simulink model "SimuModel_H_robust"  (Simulink 9.3)
settings: Solver=ode23  StartTime=0.0  StopTime=t_d  MaxStep=Tc  RelTol=1e-8  AbsTol=1e-8
values from neighbouring files (symbols this model uses):
  B_h = diag([a(1)*pi_l(1) + pi_l(2) + a(2) + pi_l(4) ... (first row only)    [InitVariable_exe.m]
  DQ = D'*Q    [InitVariable_exe.m]
  ep = 0.004    [InitVariable_exe.m]
  F_v = K_r*diag([0.01 0.01])*K_r    [InitVariable_exe.m]
  g = 9.81    [InitVariable_exe.m]
  K_d = 5*diag([1 1])    [InitVariable_exe.m]
  K_p = 25*diag([1 1])    [InitVariable_exe.m]
  q_i = [-1.4706; 2.9413]    [InitVariable_exe.m]
  rho = 70    [InitVariable_exe.m]
  Tc = 0.001    [InitVariable_exe.m]
  Ts = Tc    (= 0.001)    [InitVariable_exe.m]
undefined symbols (not defined in the file or in its folder): a, BMatrix, pi_l, pi_m
settings Model: Creator=luigivillani  LastModifiedBy=yuzg  ExtModeAutoUpdateStatusClock=off
settings SolverCC: AutoScaleAbsTol=off  InitialStep=0.1*Tc
settings DataIOCC: SaveOutput=off  SaveTime=off
settings OptimizationCC: BlockReduction=off  BooleanDataType=off  ExpressionDepthLimit=2147483647  InitFltsAndDblsToZero=on
settings DebuggingCC: SaveWithParameterizedLinksMsg=none  SignalResolutionControl=TryResolveAllWithWarning  MultiTaskDSMMsg=warning  MultiTaskCondExecSysMsg=none  StateNameClashWarn=warning
settings HardwareCC: TargetUnknown=on
settings SFSimCC: SimUseLocalCustomCode=on
settings RTWCC: RTWUseLocalCustomCode=on
settings GRTTargetCC: TargetFcnLib=ansi_tfl_tmw.mat
settings ConfigComp: CovExternalEMLEnable=on

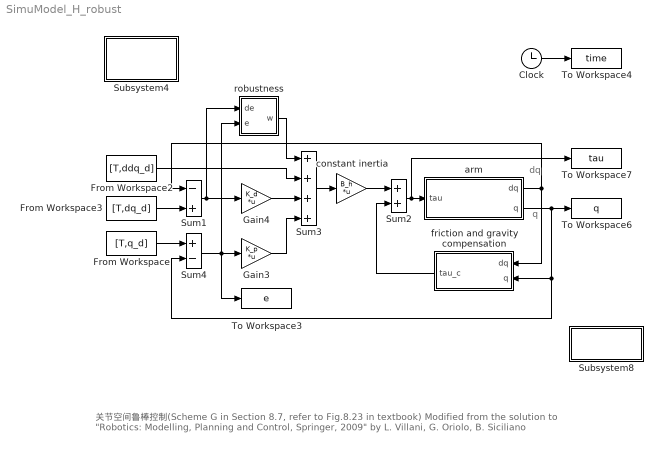
== system SimuModel_H_robust ==
  note: dq
  note: q
  note: 关节空间鲁棒控制(Scheme G in Section 8.7, refer to Fig.8.23 in textbook)
      | Modified from the solution to "Robotics: Modelling, Planning and Control, Springer, 2009" by L. Villani, G. Oriolo, B. Siciliano
  Clock : Clock
  From Workspace : FromWorkspace  VariableName=[T,q_d]  SampleTime=Tc
  From Workspace2 : FromWorkspace  VariableName=[T,ddq_d]  SampleTime=Tc
  From Workspace3 : FromWorkspace  VariableName=[T,dq_d]  SampleTime=Tc
  Gain3 : Gain  Gain=K_p  Multiplication=Matrix(K*u)  SampleTime=Tc
      mask Display: disp('K_p')
  Gain4 : Gain  Gain=K_d  Multiplication=Matrix(K*u)  SampleTime=Tc
      mask Display: disp('K_d')
  Subsystem4 : Subsystem
      settings: OpenFcn=clear all;c=0;InitVariable_exe;
      mask Display: disp('K_p = 25I\nK_d = 5I')
  Subsystem8 : Subsystem
      settings: OpenFcn=PlotFigure;
      mask Display: disp('plot')
  Sum1 : Sum  Inputs=-+  SampleTime=Tc  SaturateOnIntegerOverflow=on  InputSameDT=on  OutDataTypeStr=Inherit: Same as first input
  Sum2 : Sum  SaturateOnIntegerOverflow=on  InputSameDT=on  OutDataTypeStr=Inherit: Same as first input
  Sum3 : Sum  Inputs=++++  SaturateOnIntegerOverflow=on  InputSameDT=on  OutDataTypeStr=Inherit: Same as first input
  Sum4 : Sum  Inputs=+-  SampleTime=Tc  SaturateOnIntegerOverflow=on  InputSameDT=on  OutDataTypeStr=Inherit: Same as first input
  To Workspace3 : ToWorkspace  VariableName=e  SampleTime=Ts
      settings: MaxDataPoints=5001
  To Workspace4 : ToWorkspace  VariableName=time  SampleTime=Ts
      settings: MaxDataPoints=5001
  To Workspace6 : ToWorkspace  VariableName=q  SampleTime=Ts
      settings: MaxDataPoints=5001
  To Workspace7 : ToWorkspace  VariableName=tau  SampleTime=Ts
      settings: MaxDataPoints=5001
  arm : Subsystem
      mask Display: disp('Robot InvDynamics')
  constant inertia : Gain  Gain=B_h  Multiplication=Matrix(K*u)  SampleTime=Tc
      mask Display: disp('B_h')
  friction and gravity compensation : Subsystem
      mask Display: disp('F_vdq+g(q)')
  robustness : Subsystem
      mask Display: disp('UV')
  wires:
  Clock/1 -> To Workspace4/1
  Sum3/1 -> constant inertia/1
  friction and gravity compensation/1(tau_c) -> Sum2/2
  arm/1(dq) -> Sum1/1, friction and gravity compensation/1(dq)
  arm/2("q ") -> To Workspace6/1, friction and gravity compensation/2(q), Sum4/2
  From Workspace3/1 -> Sum1/2
  From Workspace/1 -> Sum4/1
  constant inertia/1 -> Sum2/1
  Sum4/1 -> robustness/2(e), To Workspace3/1, Gain3/1
  Sum1/1 -> robustness/1(de), Gain4/1
  Gain3/1 -> Sum3/4
  Gain4/1 -> Sum3/3
  Sum2/1 -> To Workspace7/1, arm/1(tau)
  robustness/1(w) -> Sum3/1
  From Workspace2/1 -> Sum3/2

== system SimuModel_H_robust/Subsystem4 ==
  note: start

== system SimuModel_H_robust/Subsystem8 ==
  note: start

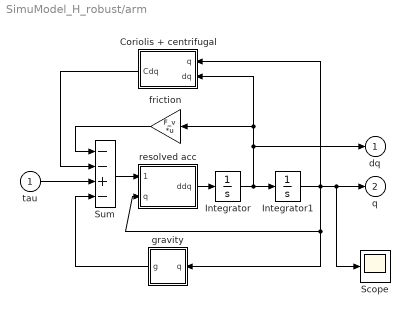
== system SimuModel_H_robust/arm ==
  tau : Inport
  Coriolis + centrifugal : Subsystem
      mask Display: disp('C(q,dq)dq')
  Integrator : Integrator  InitialCondition=[0 0]  ZeroCross=off
  Integrator1 : Integrator  InitialCondition=q_i  ZeroCross=off
  Scope : Scope
  Sum : Sum  Inputs=--+-  SaturateOnIntegerOverflow=on  InputSameDT=on  OutDataTypeStr=Inherit: Same as first input
  friction : Gain  Gain=F_v  Multiplication=Matrix(K*u)  SaturateOnIntegerOverflow=on  OutDataTypeStr=Inherit: Same as input  ParamDataTypeStr=Inherit: Same as input
      mask Display: disp('F_v')
  gravity : Subsystem
      mask Display: disp('g(q)')
  resolved acc : Subsystem
      mask Display: disp('inv(B(q))')
  dq : Outport  InitialOutput=0
  "q " : Outport  Port=2  InitialOutput=0
  wires:
  Coriolis + centrifugal/1(Cdq) -> Sum/2
  tau/1 -> Sum/3
  Integrator1/1 -> Coriolis + centrifugal/1(q), resolved acc/2(q), gravity/1(q), Scope/1, "q "/1
  resolved acc/1(ddq) -> Integrator/1
  Integrator/1 -> Integrator1/1, dq/1, Coriolis + centrifugal/2(dq), friction/1
  Sum/1 -> resolved acc/1(tau-tau')
  friction/1 -> Sum/1
  gravity/1(g) -> Sum/4

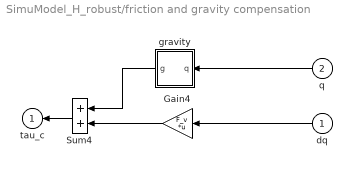
== system SimuModel_H_robust/friction and gravity compensation ==
  dq : Inport
  q : Inport  Port=2
  Gain4 : Gain  Gain=F_v  Multiplication=Matrix(K*u)  SampleTime=Tc
      mask Display: disp('F_v')
  Sum4 : Sum  SaturateOnIntegerOverflow=on  InputSameDT=on  OutDataTypeStr=Inherit: Same as first input
  gravity : Subsystem
      mask Display: disp('g(q)')
  tau_c : Outport  InitialOutput=0
  wires:
  gravity/1(g) -> Sum4/1
  Sum4/1 -> tau_c/1
  q/1 -> gravity/1(q)
  Gain4/1 -> Sum4/2
  dq/1 -> Gain4/1

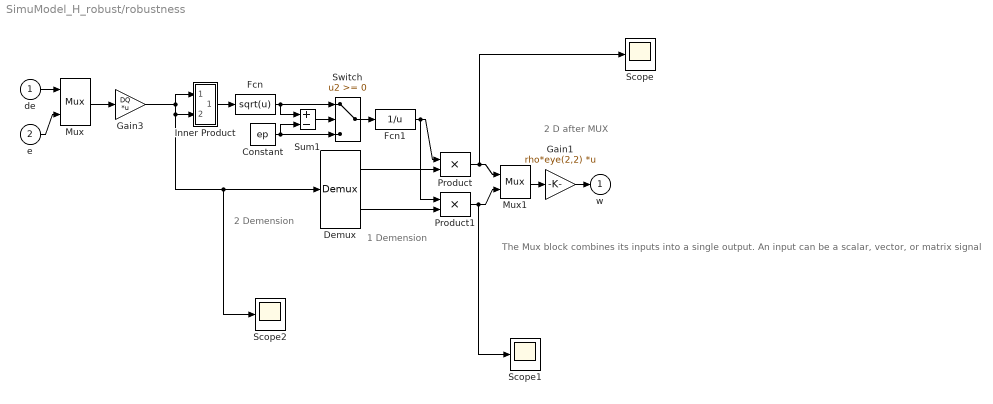
== system SimuModel_H_robust/robustness ==
  note: 2 Demension
  note: The Mux block combines its inputs into a single output. An input can be a scalar, vector, or matrix signal
  note: 1 Demension
  note: 2 D after MUX
  de : Inport
  e : Inport  Port=2
  Constant : Constant  Value=ep
  Demux : Demux  Outputs=2
  Fcn : Fcn  Expr=sqrt(u)
  Fcn1 : Fcn  Expr=1/u  SampleTime=Tc
  Gain1 : Gain  Gain=rho*eye(2,2)  Multiplication=Matrix(K*u)  SampleTime=Tc
      mask Display: disp('rho')
  Gain3 : Gain  Gain=DQ  Multiplication=Matrix(K*u)  SampleTime=Tc
      mask Display: disp('DQ')
  Inner Product : Subsystem  mask(Dot Product){}
      mask help:
      | Inner (dot) product.
      | y=sum(u1.*u2)
      mask Help: Computes the inner (dot) product of the inputs: sum(u1.*u2).  The inputs are vectors of the same length. Output is a scalar.
      mask Display: disp('.\n')
  Mux : Mux  Inputs=[2,2]
  Mux1 : Mux  Inputs=2
  Product : Product  SaturateOnIntegerOverflow=on  RndMeth=Zero  InputSameDT=on  OutDataTypeStr=Inherit: Same as first input
  Product1 : Product  SaturateOnIntegerOverflow=on  RndMeth=Zero  InputSameDT=on  OutDataTypeStr=Inherit: Same as first input
  Scope : Scope
  Scope1 : Scope
  Scope2 : Scope
  Sum1 : Sum  Inputs=+-  SaturateOnIntegerOverflow=on  InputSameDT=on  OutDataTypeStr=Inherit: Same as first input
  Switch : Switch  SaturateOnIntegerOverflow=on  InputSameDT=on
  w : Outport  InitialOutput=0
  wires:
  Demux/2 -> Product1/2
  Demux/1 -> Product/2
  Product1/1 -> Scope1/1, Mux1/2
  Product/1 -> Scope/1, Mux1/1
  Switch/1 -> Fcn1/1
  Sum1/1 -> Switch/2
  Constant/1 -> Switch/3, Sum1/2
  Fcn/1 -> Switch/1, Sum1/1
  Inner Product/1(out_1) -> Fcn/1
  de/1 -> Mux/1
  e/1 -> Mux/2
  Mux/1 -> Gain3/1
  Gain3/1 -> Inner Product/1(in_1), Inner Product/2(in_2), Scope2/1, Demux/1
  Fcn1/1 -> Product1/1, Product/1
  Mux1/1 -> Gain1/1
  Gain1/1 -> w/1

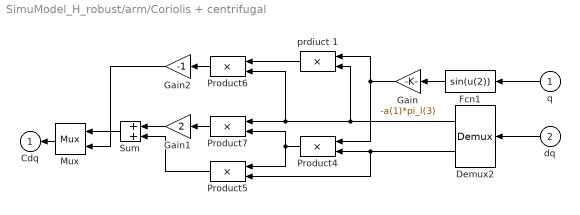
== system SimuModel_H_robust/arm/Coriolis + centrifugal ==
  q : Inport
  dq : Inport  Port=2
  Demux2 : Demux  Outputs=2
  Fcn1 : Fcn  Expr=sin(u(2))
  Gain : Gain  Gain=-a(1)*pi_l(3)  SaturateOnIntegerOverflow=on  OutDataTypeStr=Inherit: Same as input  ParamDataTypeStr=Inherit: Same as input
      mask Display: disp('k_3')
  Gain1 : Gain  Gain=2  SaturateOnIntegerOverflow=on  OutDataTypeStr=Inherit: Same as input  ParamDataTypeStr=Inherit: Same as input
  Gain2 : Gain  Gain=-1  SaturateOnIntegerOverflow=on  OutDataTypeStr=Inherit: Same as input  ParamDataTypeStr=Inherit: Same as input
  Mux : Mux  Inputs=2
  Product{4..7} (4 alike) : Product  SaturateOnIntegerOverflow=on  RndMeth=Zero  InputSameDT=on  OutDataTypeStr=Inherit: Same as first input
  Sum : Sum  SaturateOnIntegerOverflow=on  InputSameDT=on  OutDataTypeStr=Inherit: Same as first input
  prdiuct 1 : Product  SaturateOnIntegerOverflow=on  RndMeth=Zero  InputSameDT=on  OutDataTypeStr=Inherit: Same as first input
  Cdq : Outport  InitialOutput=0
  wires:
  dq/1 -> Demux2/1
  Gain2/1 -> Mux/2
  Product6/1 -> Gain2/1
  Mux/1 -> Cdq/1
  Sum/1 -> Mux/1
  Product5/1 -> Sum/2
  Gain1/1 -> Sum/1
  Product7/1 -> Gain1/1
  Demux2/1 -> prdiuct 1/2, Product6/2, Product7/1
  Demux2/2 -> Product4/2, Product5/2
  prdiuct 1/1 -> Product6/1
  Gain/1 -> prdiuct 1/1, Product4/1
  Fcn1/1 -> Gain/1
  q/1 -> Fcn1/1
  Product4/1 -> Product5/1, Product7/2

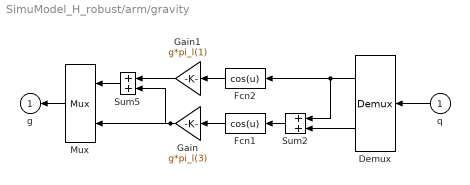
== system SimuModel_H_robust/arm/gravity ==
  q : Inport
  Demux : Demux  Outputs=2
  Fcn1 : Fcn  Expr=cos(u)
  Fcn2 : Fcn  Expr=cos(u)
  Gain : Gain  Gain=g*pi_l(3)  SaturateOnIntegerOverflow=on  OutDataTypeStr=Inherit: Same as input  ParamDataTypeStr=Inherit: Same as input
      mask Display: disp('k_2')
  Gain1 : Gain  Gain=g*pi_l(1)  SaturateOnIntegerOverflow=on  OutDataTypeStr=Inherit: Same as input  ParamDataTypeStr=Inherit: Same as input
      mask Display: disp('k_1')
  Mux : Mux  Inputs=2
  Sum2 : Sum  SaturateOnIntegerOverflow=on  InputSameDT=on  OutDataTypeStr=Inherit: Same as first input
  Sum5 : Sum  SaturateOnIntegerOverflow=on  InputSameDT=on  OutDataTypeStr=Inherit: Same as first input
  g : Outport  InitialOutput=0
  wires:
  q/1 -> Demux/1
  Demux/2 -> Sum2/2
  Sum2/1 -> Fcn1/1
  Fcn1/1 -> Gain/1
  Fcn2/1 -> Gain1/1
  Demux/1 -> Fcn2/1, Sum2/1
  Gain1/1 -> Sum5/1
  Sum5/1 -> Mux/1
  Gain/1 -> Sum5/2, Mux/2
  Mux/1 -> g/1

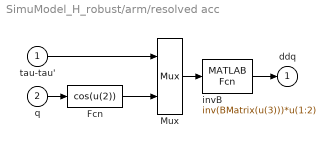
== system SimuModel_H_robust/arm/resolved acc ==
  tau-tau' : Inport
  q : Inport  Port=2
  Fcn : Fcn  Expr=cos(u(2))
  Mux : Mux  Inputs=[2,1]
  "invB " : MATLABFcn  MATLABFcn=inv(BMatrix(u(3)))*u(1:2)  OutputDimensions=2
      mask Display: disp('inv(B(q))')
  ddq : Outport  InitialOutput=0
  wires:
  Fcn/1 -> Mux/2
  q/1 -> Fcn/1
  "invB "/1 -> ddq/1
  tau-tau'/1 -> Mux/1
  Mux/1 -> "invB "/1

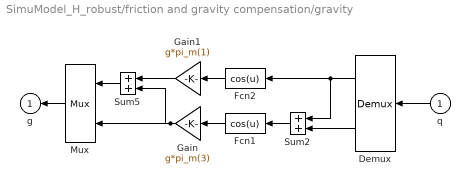
== system SimuModel_H_robust/friction and gravity compensation/gravity ==
  q : Inport
  Demux : Demux  Outputs=2
  Fcn1 : Fcn  Expr=cos(u)  SampleTime=Tc
  Fcn2 : Fcn  Expr=cos(u)  SampleTime=Tc
  Gain : Gain  Gain=g*pi_m(3)  SaturateOnIntegerOverflow=on  OutDataTypeStr=Inherit: Same as input  ParamDataTypeStr=Inherit: Same as input
      mask Display: disp('k_2')
  Gain1 : Gain  Gain=g*pi_m(1)  SaturateOnIntegerOverflow=on  OutDataTypeStr=Inherit: Same as input  ParamDataTypeStr=Inherit: Same as input
      mask Display: disp('k_1')
  Mux : Mux  Inputs=2
  Sum2 : Sum  SampleTime=Tc  SaturateOnIntegerOverflow=on  InputSameDT=on  OutDataTypeStr=Inherit: Same as first input
  Sum5 : Sum  SaturateOnIntegerOverflow=on  InputSameDT=on  OutDataTypeStr=Inherit: Same as first input
  g : Outport  InitialOutput=0
  wires:
  q/1 -> Demux/1
  Demux/2 -> Sum2/2
  Sum2/1 -> Fcn1/1
  Fcn1/1 -> Gain/1
  Fcn2/1 -> Gain1/1
  Demux/1 -> Fcn2/1, Sum2/1
  Gain1/1 -> Sum5/1
  Sum5/1 -> Mux/1
  Gain/1 -> Mux/2, Sum5/2
  Mux/1 -> g/1

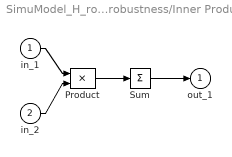
== system SimuModel_H_robust/robustness/Inner Product ==
  in_1 : Inport
  in_2 : Inport  Port=2
  Product : Product  SaturateOnIntegerOverflow=on  RndMeth=Zero  InputSameDT=on  OutDataTypeStr=Inherit: Same as first input
  Sum : Sum  Inputs=+  SaturateOnIntegerOverflow=on  InputSameDT=on  OutDataTypeStr=Inherit: Same as first input
  out_1 : Outport  InitialOutput=0
  wires:
  Sum/1 -> out_1/1
  Product/1 -> Sum/1
  in_1/1 -> Product/1
  in_2/1 -> Product/2
